simulink model "IOtoISO"  (R2017a)
settings: Solver=VariableStepAuto  StartTime=0.0  StopTime=25  MaxStep=0.01  RelTol=1e-3
settings Model: Creator=drone  LastModifiedBy=drone

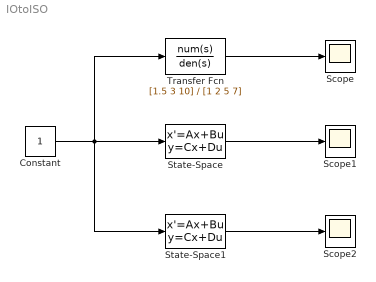
== system IOtoISO ==
  Constant : Constant
  Scope : Scope
  Scope1 : Scope
  Scope2 : Scope
  State-Space : StateSpace  A=[0 1 0; 0 0 1; -7 -5 -2;]  B=[0; 0; 1]  C=[10 3 1.5]  D=0  X0=0
  State-Space1 : StateSpace  A=[0 0 -7; 1 0 -5; 0 1 -2]  B=[10; 3; 1.5]  C=[0 0 1]  D=0  X0=0
  Transfer Fcn : TransferFcn  Numerator=[1.5 3 10]  Denominator=[1 2 5 7]
  wires:
  Constant/1 -> Transfer Fcn/1, State-Space/1, State-Space1/1
  Transfer Fcn/1 -> Scope/1
  State-Space/1 -> Scope1/1
  State-Space1/1 -> Scope2/1
